simulink model "msk"  (Simulink 5.0)
settings: Solver=ode45  StartTime=0.0  StopTime=999999  MaxStep=.025  MinStep=.00001  RelTol=1  AbsTol=1
undefined symbols (not defined in the file or in its folder): eyediasi, eyesampl, sbiterr
libraries: librnew x3
CloseFcn:
  | closemodcross
settings Model: Creator=gerhard  LastModifiedBy=bauch  ExtModeAutoUpdateStatusClock=off  SaveTime=off  SaveOutput=off  BlockReductionOpt=off  BooleanDataType=off

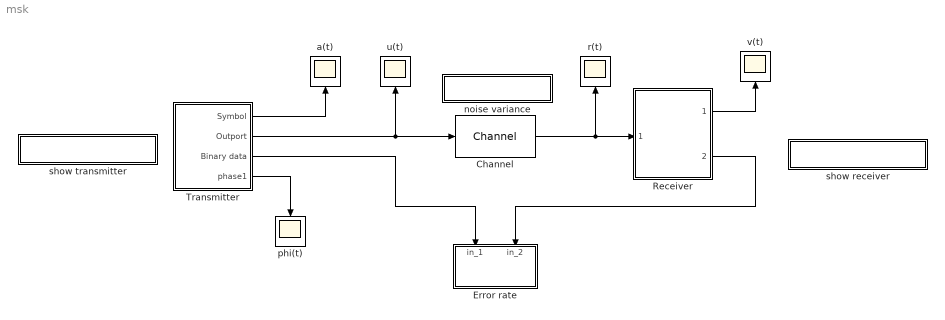
== system msk ==
  Channel : librnew/Channel  m=0  variance=0.001  s=12345
  Error rate : Subsystem  Orientation=down  LoadFcn=sbiterr([],[],[],'LoadBlock')  StartFcn=sbiterr([],[],[],'Start')  StopFcn=sbiterr([],[],[],'Stop')  mask(Symbol/bit error counter){@1=1, @2=10, @3=2, @4=1}
      mask prompts: @1 "Bit per symbol:"; @2 "Number of digits on display:"; @3 "Delay between 1st port and 2nd port:"; @4 "Sample time (sec):"
      mask help: Use the input data from the 1st port as the reference signal to detect the number of errors and error rate of the 2nd signal.
      mask init:
      | K=@1;num_lin=@2;TDelay=@3;Sample=@4;
      settings: CopyFcn=sbiterr([],[],[],'CopyBlock')  DeleteFcn=sbiterr([],[],[],'DeleteBlock')  NameChangeFcn=sbiterr([],[],[],'NameChange')
      mask Help: The signal from the first port must be a scalar. The second input port can be a vector with a delay to the first port signal. The comparison happens only at the sampling point.
      mask Display: disp('Error\nmeter')
  Receiver : Subsystem
  Transmitter : Subsystem
  a(t) : Scope
      settings: Orientation=up  TimeRange=12.500000  YMin=-3  YMax=3  DataFormat=Array
  noise variance : Subsystem
      settings: OpenFcn=setnoise
      mask Type: noise
      mask Display: disp('Noise variance')
  phi(t) : Scope
      settings: Orientation=down  TimeRange=12.500000  YMin=-3.14159  YMax=3.14159  DataFormat=Array
  r(t) : Scope
      settings: Orientation=up  TimeRange=12.500000  YMin=-1.5  YMax=1.5  DataFormat=Array
  show receiver : Subsystem
      settings: OpenFcn=showmskr
      mask Type: open
      mask Display: disp('Receiver')
  show transmitter : Subsystem
      settings: OpenFcn=showmskt
      mask Type: open
      mask Display: disp('Transmitter')
  u(t) : Scope
      settings: Orientation=up  TimeRange=12.500000  YMin=-1.5  YMax=1.5  DataFormat=Array
  v(t) : Scope
      settings: Orientation=up  TimeRange=12.500000  YMin=-3  YMax=3  DataFormat=Array
  wires:
  Transmitter/2(Outport) -> u(t)/1, Channel/1
  Channel/1 -> Receiver/1(noisy MSK signal), r(t)/1
  Transmitter/1(Symbol) -> a(t)/1
  Receiver/1(detected  symbol) -> v(t)/1
  Transmitter/4(phase1) -> phi(t)/1
  Receiver/2(detected bit) -> Error rate/2(in_2)
  Transmitter/3(Binary data) -> Error rate/1(in_1)

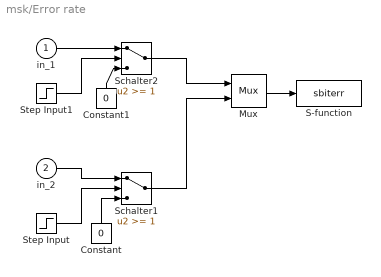
== system msk/Error rate ==
  in_1 : Inport
  in_2 : Inport  Port=2
  Constant : Constant  Orientation=up  Value=0
  Constant1 : Constant  Orientation=up  Value=0
  Mux : Mux  Inputs=2
  S-function : S-Function  FunctionName=sbiterr  Parameters=num_lin, K, TDelay, Sample
  Schalter1 : Switch  Threshold=1  SaturateOnIntegerOverflow=on  InputSameDT=on
  Schalter2 : Switch  Threshold=1  SaturateOnIntegerOverflow=on  InputSameDT=on
  Step Input : Step  Time=3  SampleTime=1
  Step Input1 : Step  SampleTime=1
  wires:
  Mux/1 -> S-function/1
  in_1/1 -> Schalter2/1
  Constant1/1 -> Schalter2/3
  Step Input1/1 -> Schalter2/2
  Schalter2/1 -> Mux/1
  in_2/1 -> Schalter1/1
  Step Input/1 -> Schalter1/2
  Constant/1 -> Schalter1/3
  Schalter1/1 -> Mux/2

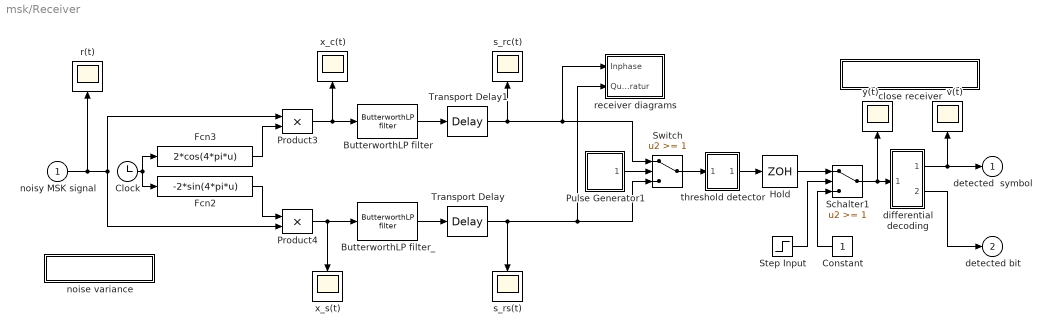
== system msk/Receiver ==
  noisy MSK signal : Inport
  ButterworthLP filter : librnew/ButterworthLP filter  n=4  MaskParam1=5
  ButterworthLP filter_ : librnew/ButterworthLP filter  n=4  MaskParam1=5
  Clock : Clock
      settings: Decimation=10
  Constant : Constant  Orientation=left
  Fcn2 : Fcn  Expr=-2*sin(4*pi*u)
  Fcn3 : Fcn  Expr=2*cos(4*pi*u)
  Hold : ZeroOrderHold
  Product3 : Product  SaturateOnIntegerOverflow=on  InputSameDT=on
  Product4 : Product  SaturateOnIntegerOverflow=on  InputSameDT=on
  Pulse Generator1 : Subsystem  mask(Pulse Generator){@1=2, @2=1, @3=1, @4=0}
      mask prompts: @1 "Pulse period (secs):"; @2 "Pulse width:"; @3 "Pulse height:"; @4 "Pulse start time:"
      mask help: Pulse Generator.
      mask init:
      | Ts=@1; du=@2; ht=@3; stt=@4; ini=ones(length(ht),1); st1=rem(stt,Ts); st2=rem(stt+du,Ts);if(Ts<=1.2*du),ini=zeros(length(ht),1);end;
      mask Help: Pulse generator which ensures pulse\ntransitions are hit. Provides a vector of pulses when the height is entered as a vector.\nUnmask to see how it works.
      mask Display: plot(0,0,100,100,[90,75,75,60,60,35,35,20,20,10],[20,20,80,80,20,20,80,80,20,20])
  Schalter1 : Switch  Threshold=1  SaturateOnIntegerOverflow=on  InputSameDT=on
  Step Input : Step  Time=2  SampleTime=1
  Switch : Switch  Threshold=1  SaturateOnIntegerOverflow=on  InputSameDT=on
  Transport Delay : TransportDelay  DelayTime=.5  BufferSize=200
  Transport Delay1 : TransportDelay  DelayTime=.5  BufferSize=200
  close receiver : Subsystem
      settings: OpenFcn=closmskr
      mask Type: close
      mask Display: disp('close receiver')
  differential decoding : Subsystem
  noise variance : Subsystem
      settings: OpenFcn=setnoise
      mask Type: noise
      mask Display: disp('Noise variance')
  r(t) : Scope
      settings: Orientation=up  TimeRange=25.000000  YMin=-2.000000  YMax=2.000000  DataFormat=Array
  receiver diagrams : Subsystem  mask(2D-Diagrams){starttime=2, anzahl=40, offset=0.075}
      mask prompts: starttime "Plot start time:"; anzahl "Samples per time slot (2*T):"; offset "Decision offset:"
      mask help: Eye pattern, signal space trajectory and scatter plot
      mask init:
      | [x, y] = srcsicon(10);
      mask Display: plot(0,0,100,100,x,y)
  s_rc(t) : Scope
      settings: Orientation=up  TimeRange=25.000000  YMin=-2.000000  YMax=2.000000  DataFormat=Array
  s_rs(t) : Scope
      settings: Orientation=down  TimeRange=25.000000  YMin=-2.000000  YMax=2.000000  DataFormat=Array
  threshold detector : Subsystem
      mask Type: Sign
      mask Description: y = sign(x)
      mask Help: Sign Function:\n\t\t\ty = 1 if x > 0\n\t\t\ty = 0 if x = 0\n\t\t\ty = -1 if x < 0
      mask Display: plot(-50,-50,50,50,[-50,50],[0,0],[0,0],[-50,50],[-40,0],[-30,-30],[0,40],[30,30])
  v(t) : Scope
      settings: Orientation=up  TimeRange=25.000000  YMin=-2.000000  YMax=2.000000  DataFormat=Array
  x_c(t) : Scope
      settings: Orientation=up  TimeRange=25.000000  YMin=-2.000000  YMax=2.000000  DataFormat=Array
  x_s(t) : Scope
      settings: Orientation=down  TimeRange=25.000000  YMin=-2.000000  YMax=2.000000  DataFormat=Array
  y(t) : Scope
      settings: Orientation=up  TimeRange=25.000000  YMin=-2.000000  YMax=2.000000  DataFormat=Array
  detected  symbol : Outport
  detected bit : Outport  Port=2
  wires:
  Fcn3/1 -> Product3/2
  Clock/1 -> Fcn3/1, Fcn2/1
  Product3/1 -> x_c(t)/1, ButterworthLP filter/1
  Product4/1 -> x_s(t)/1, ButterworthLP filter_/1
  Fcn2/1 -> Product4/1
  Pulse Generator1/1(out_1) -> Switch/2
  noisy MSK signal/1 -> r(t)/1, Product4/2, Product3/1
  differential decoding/1(out_1) -> detected  symbol/1, v(t)/1
  Switch/1 -> threshold detector/1(in_1)
  ButterworthLP filter_/1 -> Transport Delay/1
  Transport Delay/1 -> s_rs(t)/1, Switch/3, receiver diagrams/2(Quadratur)
  ButterworthLP filter/1 -> Transport Delay1/1
  Transport Delay1/1 -> s_rc(t)/1, Switch/1, receiver diagrams/1(Inphase)
  Constant/1 -> Schalter1/3
  Step Input/1 -> Schalter1/2
  threshold detector/1(out_1) -> Hold/1
  Hold/1 -> Schalter1/1
  Schalter1/1 -> differential decoding/1(in_1), y(t)/1
  differential decoding/2(Bit) -> detected bit/1

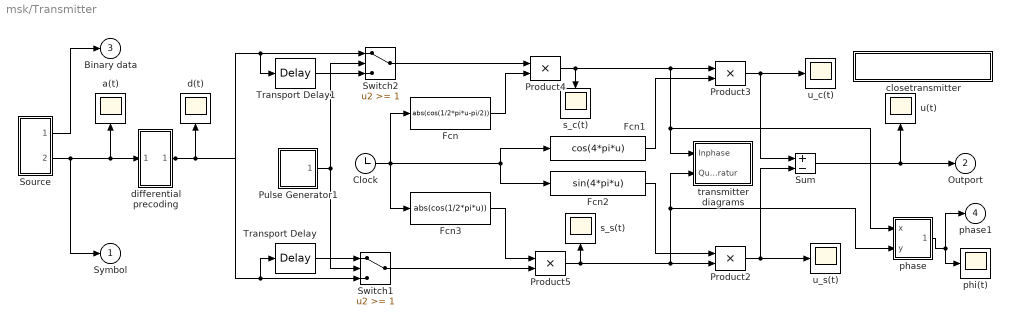
== system msk/Transmitter ==
  Clock : Clock
      settings: Decimation=10
  Fcn : Fcn  Expr=abs(cos(1/2*pi*u-pi/2))
  Fcn1 : Fcn  Expr=cos(4*pi*u)
  Fcn2 : Fcn  Expr=sin(4*pi*u)
  Fcn3 : Fcn  Expr=abs(cos(1/2*pi*u))
  Product{2..5} (4 alike) : Product  SaturateOnIntegerOverflow=on  InputSameDT=on
  Pulse Generator1 : Subsystem  mask(Pulse Generator){@1=2, @2=1, @3=1, @4=0}
      mask prompts: @1 "Pulse period (secs):"; @2 "Pulse width:"; @3 "Pulse height:"; @4 "Pulse start time:"
      mask help: Pulse Generator.
      mask init:
      | Ts=@1; du=@2; ht=@3; stt=@4; ini=ones(length(ht),1); st1=rem(stt,Ts); st2=rem(stt+du,Ts);if(Ts<=1.2*du),ini=zeros(length(ht),1);end;
      mask Help: Pulse generator which ensures pulse\ntransitions are hit. Provides a vector of pulses when the height is entered as a vector.\nUnmask to see how it works.
      mask Display: plot(0,0,100,100,[90,75,75,60,60,35,35,20,20,10],[20,20,80,80,20,20,80,80,20,20])
  Source : Subsystem
  Sum : Sum  Inputs=+-  SaturateOnIntegerOverflow=on  InputSameDT=on
  Switch1 : Switch  Threshold=1  SaturateOnIntegerOverflow=on  InputSameDT=on
  Switch2 : Switch  Threshold=1  SaturateOnIntegerOverflow=on  InputSameDT=on
  Transport Delay : TransportDelay  DelayTime=.999  BufferSize=200
  Transport Delay1 : TransportDelay  DelayTime=.999  BufferSize=200
  a(t) : Scope
      settings: Orientation=up  TimeRange=25.000000  YMin=-3.000000  YMax=3.000000  DataFormat=Array
  closetransmitter : Subsystem
      settings: OpenFcn=closmskt
      mask Type: close
      mask Display: disp('Close transmitter')
  d(t) : Scope
      settings: Orientation=up  TimeRange=12.5  YMin=-3  YMax=3  DataFormat=Array
  differential precoding : Subsystem
  phase : Subsystem
      mask Type: [x,y]->[r,theta]
      mask Description:
      | Tranformation from cartesian to polar
      | coordinates.
      | r=sqrt(x^2+y^2), theta=atan(y/x)
      mask Help: Unmask this block for more help.
      mask Display: plot(0,0,100,100,[24,20,15,20,20],[85,95,85,95,20],[80,20,95,85,95,85],[70,20,20,15,20,24],[56,56,55,52,50,46],[20,26,31,35,38,42])
  phi(t) : Scope
      settings: TimeRange=25.000000  YMin=-3.141593  YMax=3.141593  DataFormat=Array
  s_c(t) : Scope
      settings: Orientation=down  TimeRange=12.5  YMin=-1.5  YMax=1.5  DataFormat=Array
  s_s(t) : Scope
      settings: Orientation=up  TimeRange=12.5  YMin=-1.5  YMax=1.5  DataFormat=Array
  transmitter diagrams : Subsystem  mask(2D-Diagrams){starttime=1, anzahl=40, offset=0}
      mask prompts: starttime "Plot start time:"; anzahl "Samples per time slot (2*T):"; offset "Decision offset:"
      mask help: Eye pattern, signal space trajectory and scatter plot
      mask init:
      | [x, y] = srcsicon(10);
      mask Display: plot(0,0,100,100,x,y)
  u(t) : Scope
      settings: Orientation=up  TimeRange=25.000000  YMin=-1.500000  YMax=1.500000  DataFormat=Array
  u_c(t) : Scope
      settings: TimeRange=12.5  YMin=-1.5  YMax=1.5  DataFormat=Array
  u_s(t) : Scope
      settings: TimeRange=12.5  YMin=-1.5  YMax=1.5  DataFormat=Array
  Symbol : Outport
  Outport : Outport  Port=2
  Binary data : Outport  Port=3
  phase1 : Outport  Port=4
  wires:
  Sum/1 -> Outport/1, u(t)/1
  Product3/1 -> u_c(t)/1, Sum/1
  Product4/1 -> s_c(t)/1, Product3/1, transmitter diagrams/1(Inphase), phase/1(x)
  Product2/1 -> u_s(t)/1, Sum/2
  Transport Delay/1 -> Switch1/1
  differential precoding/1(out_1) -> Switch1/3, Transport Delay/1, Switch2/1, Transport Delay1/1, d(t)/1
  Clock/1 -> Fcn3/1, Fcn1/1, Fcn2/1, Fcn/1
  Switch2/1 -> Product4/1
  Switch1/1 -> Product5/2
  Transport Delay1/1 -> Switch2/3
  Fcn/1 -> Product4/2
  Fcn3/1 -> Product5/1
  Fcn1/1 -> Product3/2
  Fcn2/1 -> Product2/1
  Product5/1 -> Product2/2, transmitter diagrams/2(Quadratur), phase/2(y), s_s(t)/1
  Pulse Generator1/1(out_1) -> Switch2/2, Switch1/2
  Source/2(Symbol) -> Symbol/1, differential precoding/1(in_1), a(t)/1
  Source/1(Binärsignal) -> Binary data/1
  phase/1(theta) -> phi(t)/1, phase1/1

== system msk/noise variance ==

== system msk/show receiver ==

== system msk/show transmitter ==

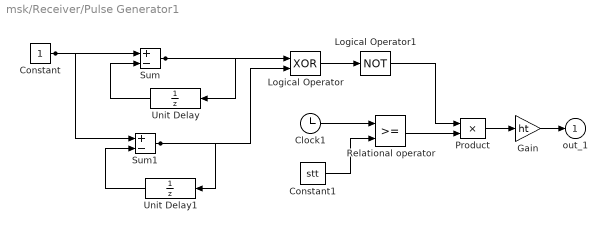
== system msk/Receiver/Pulse Generator1 ==
  Clock1 : Clock
      settings: Decimation=10
  Constant : Constant
  Constant1 : Constant  Value=stt
  Gain : Gain  Gain=ht  SaturateOnIntegerOverflow=on
  Logical Operator : Logic  Operator=XOR
  Logical Operator1 : Logic  Operator=NOT  Inputs=1
  Product : Product  SaturateOnIntegerOverflow=on  InputSameDT=on
  Relational operator : RelationalOperator  InputSameDT=on
  Sum : Sum  Inputs=+-  SaturateOnIntegerOverflow=on  InputSameDT=on
  Sum1 : Sum  Inputs=+-  SaturateOnIntegerOverflow=on  InputSameDT=on
  Unit Delay : UnitDelay  Orientation=left  SampleTime=[Ts,st1]
  Unit Delay1 : UnitDelay  Orientation=left  X0=ini  SampleTime=[Ts,st2]
  out_1 : Outport
  wires:
  Sum1/1 -> Logical Operator/2, Unit Delay1/1
  Sum/1 -> Logical Operator/1, Unit Delay/1
  Constant/1 -> Sum1/1, Sum/1
  Unit Delay1/1 -> Sum1/2
  Unit Delay/1 -> Sum/2
  Clock1/1 -> Relational operator/1
  Relational operator/1 -> Product/2
  Product/1 -> Gain/1
  Gain/1 -> out_1/1
  Constant1/1 -> Relational operator/2
  Logical Operator/1 -> Logical Operator1/1
  Logical Operator1/1 -> Product/1

== system msk/Receiver/close receiver ==

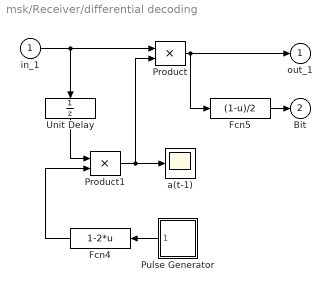
== system msk/Receiver/differential decoding ==
  in_1 : Inport
  Fcn4 : Fcn  Orientation=left  Expr=1-2*u
  Fcn5 : Fcn  Expr=(1-u)/2
  Product : Product  SaturateOnIntegerOverflow=on  InputSameDT=on
  Product1 : Product  SaturateOnIntegerOverflow=on  InputSameDT=on
  Pulse Generator : Subsystem  Orientation=left  mask(Pulse Generator){@1=2, @2=1, @3=1, @4=0}
      mask prompts: @1 "Pulse period (secs):"; @2 "Pulse width:"; @3 "Pulse height:"; @4 "Pulse start time:"
      mask help: Pulse Generator.
      mask init:
      | Ts=@1; du=@2; ht=@3; stt=@4; ini=ones(length(ht),1); st1=rem(stt,Ts); st2=rem(stt+du,Ts);if(Ts<=1.2*du),ini=zeros(length(ht),1);end;
      mask Help: Pulse generator which ensures pulse\ntransitions are hit. Provides a vector of pulses when the height is entered as a vector.\nUnmask to see how it works.
      mask Display: plot(0,0,100,100,[90,75,75,60,60,35,35,20,20,10],[20,20,80,80,20,20,80,80,20,20])
  Unit Delay : UnitDelay  Orientation=down  X0=1
  a(t-1) : Scope
      settings: TimeRange=25.000000  YMin=-1.500000  YMax=1.500000  DataFormat=Array
  out_1 : Outport
  Bit : Outport  Port=2
  wires:
  Unit Delay/1 -> Product1/1
  Product1/1 -> a(t-1)/1, Product/2
  in_1/1 -> Product/1, Unit Delay/1
  Product/1 -> out_1/1, Fcn5/1
  Pulse Generator/1(out_1) -> Fcn4/1
  Fcn4/1 -> Product1/2
  Fcn5/1 -> Bit/1

== system msk/Receiver/noise variance ==

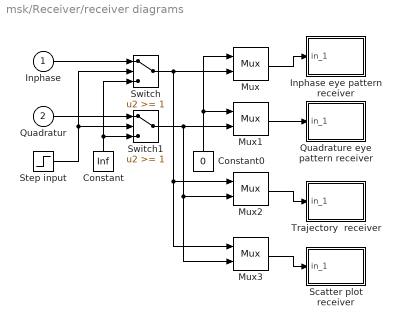
== system msk/Receiver/receiver diagrams ==
  Inphase : Inport
  Quadratur : Inport  Port=2
  Constant : Constant  Orientation=up  Value=Inf
  Constant0 : Constant  Orientation=up  Value=0
  Inphase eye pattern receiver : Subsystem  LoadFcn=eyesampl([],[],[],'LoadBlock')  StartFcn=eyesampl([],[],[],'Start')  StopFcn=eyesampl([],[],[],'Stop')  mask(Eye-diagram/scatter plot){@1=[2 0 1+offset], @2=[-1.5 1.5], @3=0, @4='w-/r-', @5=0, @6=2/anzahl}
      mask prompts: @1 "[Symbol interval, plot offset, decision point offset]:"; @2 "Lower and upper bound of in-coming signal (1x2 vector):"; @3 "Number of saved traces:"; @4 "Line-type for eye-pattern diagram (0 for no plot):"; @5 "Line-type for scatter plot (0 for no plot):"; @6 "Plot update sample time:"
      mask help: Produce eye-pattern diagram and/or scatter plot.
      mask init:
      | time_range=@1;boundary=@2;kept_length=@3;eye_line=@4;scatter_line=@5;two_d_line=@6;[x,y]=srcsicon(10);
      settings: CopyFcn=eyesampl([],[],[],'CopyBlock')  DeleteFcn=eyesampl([],[],[],'DeleteBlock')  NameChangeFcn=eyesampl([],[],[],'NameChange')
      mask Help: This plot opens one, or two plots by assigning the line type parameters. The scatter plot point is selected by the decision point in the first parameter entry. A decision line is drawn in the eye-pattern diagram. The plot is updated at the plot update sample time point.
      mask Display: plot(0,0,100,100,x,y);
  Mux{,1..3} (4 alike) : Mux  Inputs=2
  Quadrature eye pattern receiver : Subsystem  LoadFcn=eyesampl([],[],[],'LoadBlock')  StartFcn=eyesampl([],[],[],'Start')  StopFcn=eyesampl([],[],[],'Stop')  mask(Eye-diagram/scatter plot){@1=[2 0 1+offset], @2=[-1.5 1.5], @3=0, @4='w-/r-', @5=0, @6=2/anzahl}
      mask prompts: @1 "[Symbol interval, plot offset, decision point offset]:"; @2 "Lower and upper bound of in-coming signal (1x2 vector):"; @3 "Number of saved traces:"; @4 "Line-type for eye-pattern diagram (0 for no plot):"; @5 "Line-type for scatter plot (0 for no plot):"; @6 "Plot update sample time:"
      mask help: Produce eye-pattern diagram and/or scatter plot.
      mask init:
      | time_range=@1;boundary=@2;kept_length=@3;eye_line=@4;scatter_line=@5;two_d_line=@6;[x,y]=srcsicon(10);
      settings: CopyFcn=eyesampl([],[],[],'CopyBlock')  DeleteFcn=eyesampl([],[],[],'DeleteBlock')  NameChangeFcn=eyesampl([],[],[],'NameChange')
      mask Help: This plot opens one, or two plots by assigning the line type parameters. The scatter plot point is selected by the decision point in the first parameter entry. A decision line is drawn in the eye-pattern diagram. The plot is updated at the plot update sample time point.
      mask Display: plot(0,0,100,100,x,y);
  Scatter plot receiver : Subsystem  LoadFcn=eyesampl([],[],[],'LoadBlock')  StartFcn=eyesampl([],[],[],'Start')  StopFcn=eyesampl([],[],[],'Stop')  mask(Eye-diagram/scatter plot){@1=[1 .5   .999], @2=[-1.5 1.5], @3=0, @4=0, @5='b.', @6=[.5 offset]}
      mask prompts: @1 "[Symbol interval, plot offset, decision point offset]:"; @2 "Lower and upper bound of in-coming signal (1x2 vector):"; @3 "Number of saved traces:"; @4 "Line-type for eye-pattern diagram (0 for no plot):"; @5 "Line-type for scatter plot (0 for no plot):"; @6 "Plot update sample time:"
      mask help: Produce eye-pattern diagram and/or scatter plot.
      mask init:
      | time_range=@1;boundary=@2;kept_length=@3;eye_line=@4;scatter_line=@5;two_d_line=@6;[x,y]=srcsicon(10);
      settings: CopyFcn=eyesampl([],[],[],'CopyBlock')  DeleteFcn=eyesampl([],[],[],'DeleteBlock')  NameChangeFcn=eyesampl([],[],[],'NameChange')
      mask Help: This plot opens one, or two plots by assigning the line type parameters. The scatter plot point is selected by the decision point in the first parameter entry. A decision line is drawn in the eye-pattern diagram. The plot is updated at the plot update sample time point.
      mask Display: plot(0,0,100,100,x,y);
  Step input : Step  Time=starttime  SampleTime=1
  Switch : Switch  Threshold=1  SaturateOnIntegerOverflow=on  InputSameDT=on
  Switch1 : Switch  Threshold=1  SaturateOnIntegerOverflow=on  InputSameDT=on
  Trajectory  receiver : Subsystem  LoadFcn=eyediasi([],[],[],'LoadBlock')  StartFcn=eyediasi([],[],[],'Start')  StopFcn=eyediasi([],[],[],'Stop')  mask(Eye-diagram/scatter plot){@1=[2 0 1], @2=[-1.5 1.5], @3=0, @4=0, @5=0, @6='g-'}
      mask prompts: @1 "Eye-pattern plot time frame:"; @2 "Lower and upper bound of in-coming signal (1x2 vector):"; @3 "Number of saved traces:"; @4 "Line-type for eye-pattern diagram (0 for no plot):"; @5 "Line-type for scatter plot (0 for no plot):"; @6 "Line-type for x-y plot (0 for no plot):"
      mask help:
      | Produce eye-pattern diagram/scatter
      | plot/x-y plot with the rising edge of the second input as the decision line.
      mask init:
      | time_range=@1;boundary=@2;kept_length=@3;eye_line=@4;scatter_line=@5;two_d_line=@6;[x,y]=srcsicon(10);[v,w]=trigicon(0,25,get_param(gcb,'orientation'),2);
      settings: CopyFcn=eyediasi([],[],[],'CopyBlock')  DeleteFcn=eyediasi([],[],[],'DeleteBlock')  NameChangeFcn=eyediasi([],[],[],'NameChange')
      mask Help: This plot opens one, two, or three plots by assigning the line type parameters. The scatter plot point is selected by the rising edge of a trigger signal. A decision line is drawn at the rising edge of the trigger signal.
      mask Display: plot(0,0,100,100,x,y,v,w);
  wires:
  Switch/1 -> Mux2/1, Mux3/1, Mux/2
  Switch1/1 -> Mux2/2, Mux3/2, Mux1/2
  Constant0/1 -> Mux1/1, Mux/1
  Quadratur/1 -> Switch1/1
  Inphase/1 -> Switch/1
  Step input/1 -> Switch/2, Switch1/2
  Constant/1 -> Switch/3, Switch1/3
  Mux1/1 -> Quadrature eye pattern receiver/1(in_1)
  Mux/1 -> Inphase eye pattern receiver/1(in_1)
  Mux3/1 -> Scatter plot receiver/1(in_1)
  Mux2/1 -> Trajectory  receiver/1(in_1)

== system msk/Receiver/threshold detector ==
  in_1 : Inport
  Constant : Constant  Value=0
  Relational Operator : RelationalOperator  Operator=>  InputSameDT=on
  Relational Operator1 : RelationalOperator  Operator=<  InputSameDT=on
  Sum : Sum  Inputs=+-  SaturateOnIntegerOverflow=on  InputSameDT=on
  out_1 : Outport
  wires:
  in_1/1 -> Relational Operator/1, Relational Operator1/1
  Constant/1 -> Relational Operator1/2, Relational Operator/2
  Relational Operator1/1 -> Sum/2
  Relational Operator/1 -> Sum/1
  Sum/1 -> out_1/1

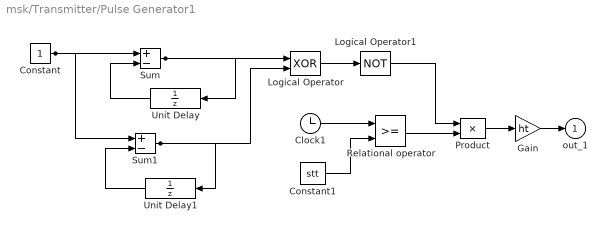
== system msk/Transmitter/Pulse Generator1 ==
  Clock1 : Clock
      settings: Decimation=10
  Constant : Constant
  Constant1 : Constant  Value=stt
  Gain : Gain  Gain=ht  SaturateOnIntegerOverflow=on
  Logical Operator : Logic  Operator=XOR
  Logical Operator1 : Logic  Operator=NOT  Inputs=1
  Product : Product  SaturateOnIntegerOverflow=on  InputSameDT=on
  Relational operator : RelationalOperator  InputSameDT=on
  Sum : Sum  Inputs=+-  SaturateOnIntegerOverflow=on  InputSameDT=on
  Sum1 : Sum  Inputs=+-  SaturateOnIntegerOverflow=on  InputSameDT=on
  Unit Delay : UnitDelay  Orientation=left  SampleTime=[Ts,st1]
  Unit Delay1 : UnitDelay  Orientation=left  X0=ini  SampleTime=[Ts,st2]
  out_1 : Outport
  wires:
  Logical Operator1/1 -> Product/1
  Logical Operator/1 -> Logical Operator1/1
  Constant1/1 -> Relational operator/2
  Gain/1 -> out_1/1
  Product/1 -> Gain/1
  Relational operator/1 -> Product/2
  Clock1/1 -> Relational operator/1
  Unit Delay/1 -> Sum/2
  Sum/1 -> Unit Delay/1, Logical Operator/1
  Constant/1 -> Sum/1, Sum1/1
  Sum1/1 -> Unit Delay1/1, Logical Operator/2
  Unit Delay1/1 -> Sum1/2

== system msk/Transmitter/Source ==
  Fcn : Fcn  Expr=1-2*u
  Source : Subsystem  mask(Read from workspace){@1=randint(1000,1,2), @2=1, @3=1, @4=1}
      mask prompts: @1 "Variable (column_number=block_output_length):"; @2 "Data output sample time (sec):"; @3 "Repeat flag (1: repeat read, 0: output zeros after eof)."; @4 "Initial output:"
      mask help:
      | Read from a workspace variable at
      | sampling time point.
      mask init:
      | var=@1;td=@2;ts=td(1);if (length(td)>=2),off=td(2);else off=0;end;cyc=@3;ini=@4;[x,y]=srcsicon(7);
      mask Help: This block reads from a workspace variable at a given sample time. The column number is the block output vector length. When the simulation reaches the end of the variable (eof), the block will cyclically output from the first row of the variable or output zeros based on the repeat flag entree.
      mask Display: plot(0,0,100,100,x,y);disp('Rd wksp')
  Binärsignal : Outport
  Symbol : Outport  Port=2
  wires:
  Source/1(out_1) -> Fcn/1, Binärsignal/1
  Fcn/1 -> Symbol/1

== system msk/Transmitter/closetransmitter ==

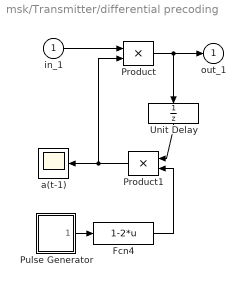
== system msk/Transmitter/differential precoding ==
  in_1 : Inport
  Fcn4 : Fcn  Expr=1-2*u
  Product : Product  SaturateOnIntegerOverflow=on  InputSameDT=on
  Product1 : Product  Orientation=left  SaturateOnIntegerOverflow=on  InputSameDT=on
  Pulse Generator : Subsystem  mask(Pulse Generator){@1=2, @2=1, @3=1, @4=0}
      mask prompts: @1 "Pulse period (secs):"; @2 "Pulse width:"; @3 "Pulse height:"; @4 "Pulse start time:"
      mask help: Pulse Generator.
      mask init:
      | Ts=@1; du=@2; ht=@3; stt=@4; ini=ones(length(ht),1); st1=rem(stt,Ts); st2=rem(stt+du,Ts);if(Ts<=1.2*du),ini=zeros(length(ht),1);end;
      mask Help: Pulse generator which ensures pulse\ntransitions are hit. Provides a vector of pulses when the height is entered as a vector.\nUnmask to see how it works.
      mask Display: plot(0,0,100,100,[90,75,75,60,60,35,35,20,20,10],[20,20,80,80,20,20,80,80,20,20])
  Unit Delay : UnitDelay  Orientation=down  X0=1
  a(t-1) : Scope
      settings: TimeRange=25.000000  YMin=-1.500000  YMax=1.500000  DataFormat=Array
  out_1 : Outport
  wires:
  Product1/1 -> a(t-1)/1, Product/2
  Product/1 -> out_1/1, Unit Delay/1
  in_1/1 -> Product/1
  Unit Delay/1 -> Product1/1
  Pulse Generator/1(out_1) -> Fcn4/1
  Fcn4/1 -> Product1/2

== system msk/Transmitter/phase ==
  note: Cartesian to Polar
  x : Inport
  y : Inport  Port=2
  Mux : Mux  Inputs=2
  Terminator : Terminator
  x->r : Fcn  Expr=hypot(u[1],u[2])
  x->theta : Fcn  Expr=atan2(u[2],u[1])
  theta : Outport
  wires:
  x->theta/1 -> theta/1
  y/1 -> Mux/2
  x/1 -> Mux/1
  x->r/1 -> Terminator/1
  Mux/1 -> x->r/1, x->theta/1

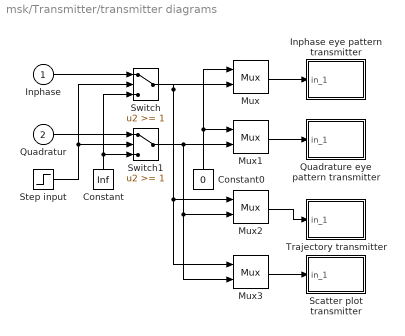
== system msk/Transmitter/transmitter diagrams ==
  Inphase : Inport
  Quadratur : Inport  Port=2
  Constant : Constant  Orientation=up  Value=Inf
  Constant0 : Constant  Orientation=up  Value=0
  Inphase eye pattern transmitter : Subsystem  LoadFcn=eyesampl([],[],[],'LoadBlock')  StartFcn=eyesampl([],[],[],'Start')  StopFcn=eyesampl([],[],[],'Stop')  mask(Eye-diagram/scatter plot){@1=[2 0 1+offset], @2=[-1.5 1.5], @3=0, @4='w-/r-', @5=0, @6=2/anzahl}
      mask prompts: @1 "[Symbol interval, plot offset, decision point offset]:"; @2 "Lower and upper bound of in-coming signal (1x2 vector):"; @3 "Number of saved traces:"; @4 "Line-type for eye-pattern diagram (0 for no plot):"; @5 "Line-type for scatter plot (0 for no plot):"; @6 "Plot update sample time:"
      mask help: Produce eye-pattern diagram and/or scatter plot.
      mask init:
      | time_range=@1;boundary=@2;kept_length=@3;eye_line=@4;scatter_line=@5;two_d_line=@6;[x,y]=srcsicon(10);
      settings: CopyFcn=eyesampl([],[],[],'CopyBlock')  DeleteFcn=eyesampl([],[],[],'DeleteBlock')  NameChangeFcn=eyesampl([],[],[],'NameChange')
      mask Help: This plot opens one, or two plots by assigning the line type parameters. The scatter plot point is selected by the decision point in the first parameter entry. A decision line is drawn in the eye-pattern diagram. The plot is updated at the plot update sample time point.
      mask Display: plot(0,0,100,100,x,y);
  Mux{,1..3} (4 alike) : Mux  Inputs=2
  Quadrature eye pattern transmitter : Subsystem  LoadFcn=eyesampl([],[],[],'LoadBlock')  StartFcn=eyesampl([],[],[],'Start')  StopFcn=eyesampl([],[],[],'Stop')  mask(Eye-diagram/scatter plot){@1=[2 0 1+offset], @2=[-1.5 1.5], @3=0, @4='w-/r-', @5=0, @6=2/anzahl}
      mask prompts: @1 "[Symbol interval, plot offset, decision point offset]:"; @2 "Lower and upper bound of in-coming signal (1x2 vector):"; @3 "Number of saved traces:"; @4 "Line-type for eye-pattern diagram (0 for no plot):"; @5 "Line-type for scatter plot (0 for no plot):"; @6 "Plot update sample time:"
      mask help: Produce eye-pattern diagram and/or scatter plot.
      mask init:
      | time_range=@1;boundary=@2;kept_length=@3;eye_line=@4;scatter_line=@5;two_d_line=@6;[x,y]=srcsicon(10);
      settings: CopyFcn=eyesampl([],[],[],'CopyBlock')  DeleteFcn=eyesampl([],[],[],'DeleteBlock')  NameChangeFcn=eyesampl([],[],[],'NameChange')
      mask Help: This plot opens one, or two plots by assigning the line type parameters. The scatter plot point is selected by the decision point in the first parameter entry. A decision line is drawn in the eye-pattern diagram. The plot is updated at the plot update sample time point.
      mask Display: plot(0,0,100,100,x,y);
  Scatter plot transmitter : Subsystem  LoadFcn=eyesampl([],[],[],'LoadBlock')  StartFcn=eyesampl([],[],[],'Start')  StopFcn=eyesampl([],[],[],'Stop')  mask(Eye-diagram/scatter plot){@1=[1 .5 .999], @2=[-1.5 1.5], @3=0, @4=0, @5='b.', @6=[.5 offset]}
      mask prompts: @1 "[Symbol interval, plot offset, decision point offset]:"; @2 "Lower and upper bound of in-coming signal (1x2 vector):"; @3 "Number of saved traces:"; @4 "Line-type for eye-pattern diagram (0 for no plot):"; @5 "Line-type for scatter plot (0 for no plot):"; @6 "Plot update sample time:"
      mask help: Produce eye-pattern diagram and/or scatter plot.
      mask init:
      | time_range=@1;boundary=@2;kept_length=@3;eye_line=@4;scatter_line=@5;two_d_line=@6;[x,y]=srcsicon(10);
      settings: CopyFcn=eyesampl([],[],[],'CopyBlock')  DeleteFcn=eyesampl([],[],[],'DeleteBlock')  NameChangeFcn=eyesampl([],[],[],'NameChange')
      mask Help: This plot opens one, or two plots by assigning the line type parameters. The scatter plot point is selected by the decision point in the first parameter entry. A decision line is drawn in the eye-pattern diagram. The plot is updated at the plot update sample time point.
      mask Display: plot(0,0,100,100,x,y);
  Step input : Step  Time=starttime  SampleTime=1
  Switch : Switch  Threshold=1  SaturateOnIntegerOverflow=on  InputSameDT=on
  Switch1 : Switch  Threshold=1  SaturateOnIntegerOverflow=on  InputSameDT=on
  Trajectory transmitter : Subsystem  LoadFcn=eyediasi([],[],[],'LoadBlock')  StartFcn=eyediasi([],[],[],'Start')  StopFcn=eyediasi([],[],[],'Stop')  mask(Eye-diagram/scatter plot){@1=[2 0 1], @2=[-1.5 1.5], @3=0, @4=0, @5=0, @6='g-'}
      mask prompts: @1 "Eye-pattern plot time frame:"; @2 "Lower and upper bound of in-coming signal (1x2 vector):"; @3 "Number of saved traces:"; @4 "Line-type for eye-pattern diagram (0 for no plot):"; @5 "Line-type for scatter plot (0 for no plot):"; @6 "Line-type for x-y plot (0 for no plot):"
      mask help:
      | Produce eye-pattern diagram/scatter
      | plot/x-y plot with the rising edge of the second input as the decision line.
      mask init:
      | time_range=@1;boundary=@2;kept_length=@3;eye_line=@4;scatter_line=@5;two_d_line=@6;[x,y]=srcsicon(10);[v,w]=trigicon(0,25,get_param(gcb,'orientation'),2);
      settings: CopyFcn=eyediasi([],[],[],'CopyBlock')  DeleteFcn=eyediasi([],[],[],'DeleteBlock')  NameChangeFcn=eyediasi([],[],[],'NameChange')
      mask Help: This plot opens one, two, or three plots by assigning the line type parameters. The scatter plot point is selected by the rising edge of a trigger signal. A decision line is drawn at the rising edge of the trigger signal.
      mask Display: plot(0,0,100,100,x,y,v,w);
  wires:
  Mux2/1 -> Trajectory transmitter/1(in_1)
  Mux3/1 -> Scatter plot transmitter/1(in_1)
  Mux/1 -> Inphase eye pattern transmitter/1(in_1)
  Mux1/1 -> Quadrature eye pattern transmitter/1(in_1)
  Constant/1 -> Switch/3, Switch1/3
  Step input/1 -> Switch/2, Switch1/2
  Inphase/1 -> Switch/1
  Quadratur/1 -> Switch1/1
  Switch/1 -> Mux3/1, Mux2/1, Mux/2
  Switch1/1 -> Mux3/2, Mux2/2, Mux1/2
  Constant0/1 -> Mux1/1, Mux/1

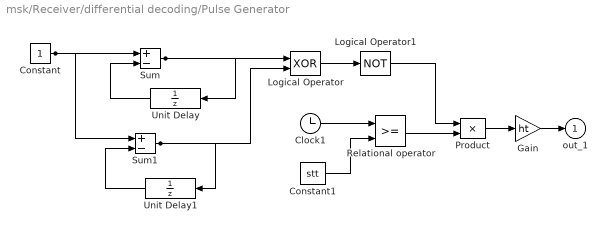
== system msk/Receiver/differential decoding/Pulse Generator ==
  Clock1 : Clock
      settings: Decimation=10
  Constant : Constant
  Constant1 : Constant  Value=stt
  Gain : Gain  Gain=ht  SaturateOnIntegerOverflow=on
  Logical Operator : Logic  Operator=XOR
  Logical Operator1 : Logic  Operator=NOT  Inputs=1
  Product : Product  SaturateOnIntegerOverflow=on  InputSameDT=on
  Relational operator : RelationalOperator  InputSameDT=on
  Sum : Sum  Inputs=+-  SaturateOnIntegerOverflow=on  InputSameDT=on
  Sum1 : Sum  Inputs=+-  SaturateOnIntegerOverflow=on  InputSameDT=on
  Unit Delay : UnitDelay  Orientation=left  SampleTime=[Ts,st1]
  Unit Delay1 : UnitDelay  Orientation=left  X0=ini  SampleTime=[Ts,st2]
  out_1 : Outport
  wires:
  Logical Operator1/1 -> Product/1
  Logical Operator/1 -> Logical Operator1/1
  Constant1/1 -> Relational operator/2
  Gain/1 -> out_1/1
  Product/1 -> Gain/1
  Relational operator/1 -> Product/2
  Clock1/1 -> Relational operator/1
  Unit Delay/1 -> Sum/2
  Sum/1 -> Unit Delay/1, Logical Operator/1
  Constant/1 -> Sum/1, Sum1/1
  Sum1/1 -> Unit Delay1/1, Logical Operator/2
  Unit Delay1/1 -> Sum1/2

== system msk/Receiver/receiver diagrams/Inphase eye pattern receiver ==
  in_1 : Inport
  Plot1 : S-Function  FunctionName=eyesampl  Parameters=time_range, boundary, kept_length, eye_line, scatter_line, two_d_line
  wires:
  in_1/1 -> Plot1/1

== system msk/Receiver/receiver diagrams/Quadrature eye pattern receiver ==
  in_1 : Inport
  Plot1 : S-Function  FunctionName=eyesampl  Parameters=time_range, boundary, kept_length, eye_line, scatter_line, two_d_line
  wires:
  in_1/1 -> Plot1/1

== system msk/Receiver/receiver diagrams/Scatter plot receiver ==
  in_1 : Inport
  Plot1 : S-Function  FunctionName=eyesampl  Parameters=time_range, boundary, kept_length, eye_line, scatter_line, two_d_line
  wires:
  in_1/1 -> Plot1/1

== system msk/Receiver/receiver diagrams/Trajectory  receiver ==
  in_1 : Inport
  Constant : Constant  Value=0
  Mux : Mux  Inputs=2
  Plot1 : S-Function  FunctionName=eyediasi  Parameters=time_range, boundary, kept_length, eye_line, scatter_line, two_d_line
  wires:
  in_1/1 -> Mux/1
  Constant/1 -> Mux/2
  Mux/1 -> Plot1/1

== system msk/Transmitter/Source/Source ==
  Message source : S-Function  FunctionName=trigwksp  Parameters=var,thd,cyclFlag,ini  mask(Read from workspace){@1=var, @2=.1, @3=cyc, @4=ini}
      mask prompts: @1 "Read the variable:"; @2 "Threshold for the input pulse:"; @3 "Cyclic read variable (1) or amend zeros (0)."; @4 "Output before first trigger:"
      mask help: The raising edge of input pulse trigger the block output the next row from the workspace variable.
      mask init:
      | var=@1;thd=@2;cyclFlag=@3;ini=@4;
      mask Help: This block reads the data from a workspace variable. The output is refreshed at the raising edge of the input pulse.
      mask Display: disp('Triggered\nread')
  Pulses deivide same sample time1 : Subsystem  mask(Pulse generator){@1=ts, @2=1, @3=off}
      mask prompts: @1 "Sample time (scalar, sec):"; @2 "Divider (integer vector):"; @3 "Offset (have same dimension as Divider:"
      mask help: Vector pulses with sample rate of each pulse as Sample_time ./Divider.
      mask init:
      | samp_time=@1;out_divid=@2;offset=@3;
      mask Help: This block generator a vector pulses. The output length is the same as the vector defined in "Divider". The ith element of the output has the sample time Sample_time/Divider(i). All elements in "Divider" must be integers.
      mask Display: disp('Vector\nPulse')
  out_1 : Outport
  wires:
  Pulses deivide same sample time1/1(Outport) -> Message source/1
  Message source/1 -> out_1/1

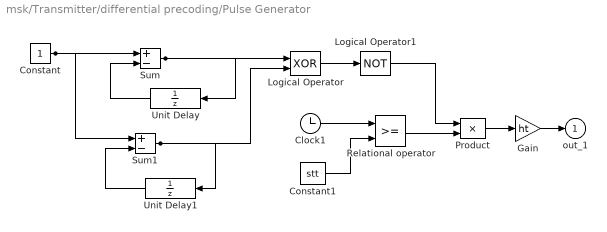
== system msk/Transmitter/differential precoding/Pulse Generator ==
  Clock1 : Clock
      settings: Decimation=10
  Constant : Constant
  Constant1 : Constant  Value=stt
  Gain : Gain  Gain=ht  SaturateOnIntegerOverflow=on
  Logical Operator : Logic  Operator=XOR
  Logical Operator1 : Logic  Operator=NOT  Inputs=1
  Product : Product  SaturateOnIntegerOverflow=on  InputSameDT=on
  Relational operator : RelationalOperator  InputSameDT=on
  Sum : Sum  Inputs=+-  SaturateOnIntegerOverflow=on  InputSameDT=on
  Sum1 : Sum  Inputs=+-  SaturateOnIntegerOverflow=on  InputSameDT=on
  Unit Delay : UnitDelay  Orientation=left  SampleTime=[Ts,st1]
  Unit Delay1 : UnitDelay  Orientation=left  X0=ini  SampleTime=[Ts,st2]
  out_1 : Outport
  wires:
  Sum1/1 -> Logical Operator/2, Unit Delay1/1
  Sum/1 -> Logical Operator/1, Unit Delay/1
  Constant/1 -> Sum1/1, Sum/1
  Unit Delay1/1 -> Sum1/2
  Unit Delay/1 -> Sum/2
  Clock1/1 -> Relational operator/1
  Relational operator/1 -> Product/2
  Product/1 -> Gain/1
  Gain/1 -> out_1/1
  Constant1/1 -> Relational operator/2
  Logical Operator/1 -> Logical Operator1/1
  Logical Operator1/1 -> Product/1

== system msk/Transmitter/transmitter diagrams/Inphase eye pattern transmitter ==
  in_1 : Inport
  Plot1 : S-Function  FunctionName=eyesampl  Parameters=time_range, boundary, kept_length, eye_line, scatter_line, two_d_line
  wires:
  in_1/1 -> Plot1/1

== system msk/Transmitter/transmitter diagrams/Quadrature eye pattern transmitter ==
  in_1 : Inport
  Plot1 : S-Function  FunctionName=eyesampl  Parameters=time_range, boundary, kept_length, eye_line, scatter_line, two_d_line
  wires:
  in_1/1 -> Plot1/1

== system msk/Transmitter/transmitter diagrams/Scatter plot transmitter ==
  in_1 : Inport
  Plot1 : S-Function  FunctionName=eyesampl  Parameters=time_range, boundary, kept_length, eye_line, scatter_line, two_d_line
  wires:
  in_1/1 -> Plot1/1

== system msk/Transmitter/transmitter diagrams/Trajectory transmitter ==
  in_1 : Inport
  Constant : Constant  Value=0
  Mux : Mux  Inputs=2
  Plot1 : S-Function  FunctionName=eyediasi  Parameters=time_range, boundary, kept_length, eye_line, scatter_line, two_d_line
  wires:
  Mux/1 -> Plot1/1
  Constant/1 -> Mux/2
  in_1/1 -> Mux/1

== system msk/Transmitter/Source/Source/Pulses deivide same sample time1 ==
  S-function1 : S-Function  FunctionName=homopuls  Parameters=samp_time, out_divid, offset
  Outport : Outport
  wires:
  S-function1/1 -> Outport/1
